simulink model "Saturation_subsystem"  (R2022b)
settings: Solver=FixedStepAuto  StartTime=0.0  StopTime=10.0  FixedStep=1e-3  RelTol=1e-3
settings Model: Creator=Abanob_Sameh  LastModifiedBy=Abanob_Sameh

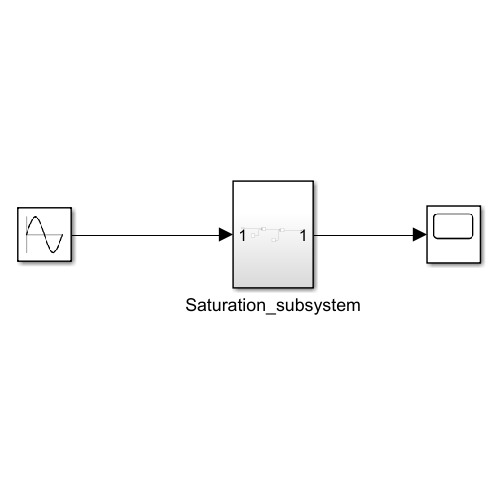
[thumbnail: Simulink's stored preview of the top-level diagram]
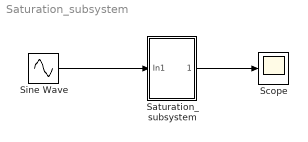
== system Saturation_subsystem ==
  Saturation_subsystem : Subsystem
  Scope : Scope
  Sine Wave : Sin  SampleTime=0
  wires:
  Sine Wave/1 -> Saturation_subsystem/1(In1)
  Saturation_subsystem/1(Out1) -> Scope/1

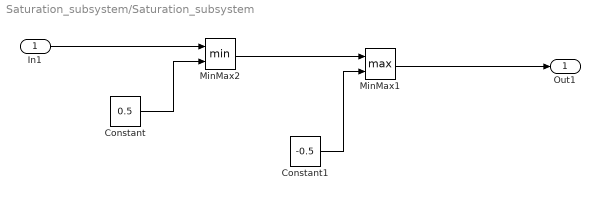
== system Saturation_subsystem/Saturation_subsystem ==
  In1 : Inport
  Constant : Constant  Value=0.5
  Constant1 : Constant  Value=-0.5
  MinMax1 : MinMax  Function=max  Inputs=2
  MinMax2 : MinMax  Inputs=2
  Out1 : Outport
  wires:
  Constant1/1 -> MinMax1/2
  Constant/1 -> MinMax2/2
  MinMax2/1 -> MinMax1/1
  MinMax1/1 -> Out1/1
  In1/1 -> MinMax2/1
